simulink model "dynamicDecouplingControl"  (R2017b)
settings: Solver=VariableStepAuto  StartTime=0.0  StopTime=time  RelTol=1e-3
values from neighbouring files (symbols this model uses):
  Kp = eye(2)    [runDynamic.m]    (also in runStatic.m)
  Kv = eye(2)    [runDynamic.m]
  L = 0.13    [runDynamic.m]    (also in runLyapunov.m; runStatic.m)
  L_controller = 0.13    [runDynamic.m]    (also in runLyapunov.m = 0.143; runStatic.m)
  R = 2    [runDynamic.m]    (also in runLyapunov.m; runStatic.m)
  r = 0.1    [runDynamic.m]    (also in runLyapunov.m; runStatic.m)
  r_controller = 0.1    [runDynamic.m]    (also in runLyapunov.m; runStatic.m)
  satMax = inf    [runDynamic.m]    (also in runLyapunov.m; runStatic.m)
  satMin = -inf    [runDynamic.m]    (also in runLyapunov.m; runStatic.m)
  wd = 0.5    [runDynamic.m]    (also in runLyapunov.m; runStatic.m)
  Xi = [2.3; 0; pi]    [runDynamic.m]    (also in runLyapunov.m; runStatic.m)
settings Model: Creator=yleni  LastModifiedBy=yleni

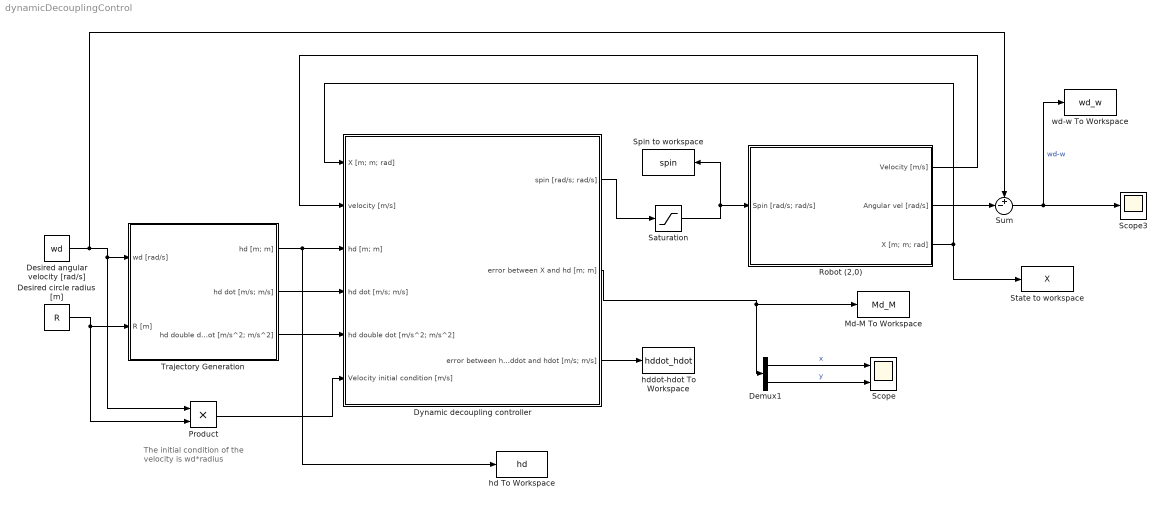
== system dynamicDecouplingControl ==
  note: The initial condition of the
      | velocity is wd*radius
  Demux1 : Demux  Outputs=2
  Desired angular velocity [rad/s] : Constant  Value=wd
  Desired circle radius [m] : Constant  Value=R
  Dynamic decoupling controller : Subsystem  mask{Kp=Kp, Kv=Kv, L=L_controller, r=r_controller}
      mask prompts: Kp "Gain position control law"; Kv "Gain velocity control law"; L "Distance from the wheel to the robot frame center [m]"; r "Wheel radius [m]"
      settings: MinAlgLoopOccurrences=on
  Md-M To Workspace : ToWorkspace  VariableName=Md_M  SampleTime=-1
      settings: Save2DSignal=2-D array (concatenate along first dimension)
  Product : Product
  Robot (2,0) : Subsystem  mask{r=r, L=L, Xstart=Xi}
      mask prompts: r "Wheel radius [m]"; L "Distance from the wheel to the robot frame center [m]"; Xstart "Initial conditions [m; m; rad]"
  Saturation : Saturate  UpperLimit=satMax  LowerLimit=satMin
  Scope : Scope  NumInputPorts=2
  Scope3 : Scope
  Spin to workspace : ToWorkspace  VariableName=spin  SampleTime=-1
      settings: Save2DSignal=2-D array (concatenate along first dimension)
  State to workspace : ToWorkspace  VariableName=X  SampleTime=-1
      settings: Save2DSignal=2-D array (concatenate along first dimension)
  Sum : Sum  Inputs=+-|
  Trajectory Generation : Subsystem
  hd To Workspace : ToWorkspace  VariableName=hd  SampleTime=-1
      settings: Save2DSignal=2-D array (concatenate along first dimension)
  hddot-hdot To Workspace : ToWorkspace  VariableName=hddot_hdot  SampleTime=-1
      settings: Save2DSignal=2-D array (concatenate along first dimension)
  wd-w To Workspace : ToWorkspace  VariableName=wd_w  SampleTime=-1
      settings: Save2DSignal=2-D array (concatenate along first dimension)
  wires:
  Robot (2,0)/3(X [m; m; rad]) -> State to workspace/1, Dynamic decoupling controller/1(X [m; m; rad])
  Desired circle radius [m]/1 -> Product/2, Trajectory Generation/2(R [m])
  Trajectory Generation/1(hd [m; m]) -> hd To Workspace/1, Dynamic decoupling controller/3(hd [m; m])
  Trajectory Generation/2(hd dot [m/s; m/s]) -> Dynamic decoupling controller/4(hd dot [m/s; m/s])
  Trajectory Generation/3(hd double dot [m/s^2; m/s^2]) -> Dynamic decoupling controller/5(hd double dot [m/s^2; m/s^2])
  Dynamic decoupling controller/1(spin [rad/s; rad/s]) -> Saturation/1
  Product/1 -> Dynamic decoupling controller/6(Velocity initial condition [m/s])
  Demux1/2 -> Scope/2  "y"
  Dynamic decoupling controller/2(error between X and hd [m; m]) -> Md-M To Workspace/1, Demux1/1
  Demux1/1 -> Scope/1  "x"
  Desired angular velocity [rad/s]/1 -> Sum/1, Product/1, Trajectory Generation/1(wd [rad/s])
  Sum/1 -> wd-w To Workspace/1, Scope3/1  "wd-w"
  Robot (2,0)/2(Angular vel [rad/s]) -> Sum/2
  Saturation/1 -> Spin to workspace/1, Robot (2,0)/1(Spin [rad/s; rad/s])
  Dynamic decoupling controller/3(error between hddot and hdot [m/s; m/s]) -> hddot-hdot To Workspace/1
  Robot (2,0)/1(Velocity [m/s]) -> Dynamic decoupling controller/2(velocity [m/s])

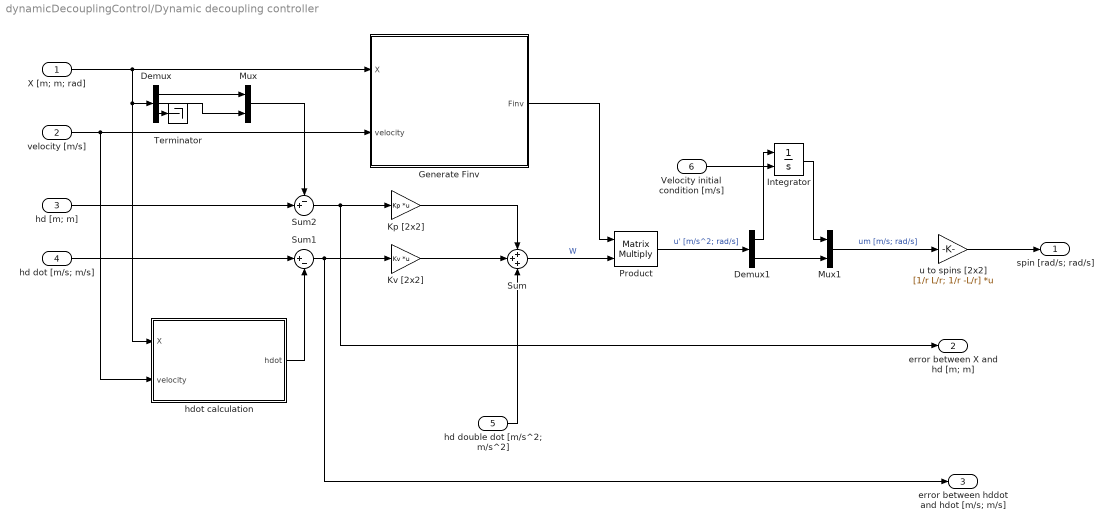
== system dynamicDecouplingControl/Dynamic decoupling controller ==
  X [m; m; rad] : Inport
  velocity [m/s] : Inport  Port=2
  hd [m; m] : Inport  Port=3
  hd dot [m/s; m/s] : Inport  Port=4
  hd double dot [m/s^2; m/s^2] : Inport  Port=5
  Velocity initial condition [m/s] : Inport  Port=6
  Demux : Demux  Outputs=3
  Demux1 : Demux  Outputs=2
  Generate Finv : MATLAB Function  TreatAsAtomicUnit=on
  Integrator : Integrator  InitialConditionSource=external
  Kp [2x2] : Gain  Gain=Kp  Multiplication=Matrix(K*u)
  Kv [2x2] : Gain  Gain=Kv  Multiplication=Matrix(K*u)
  Mux : Mux  Inputs=2
  Mux1 : Mux  Inputs=2
  Product : Product  Multiplication=Matrix(*)
  Sum : Sum  Inputs=+++
  Sum1 : Sum  Inputs=|+-
  Sum2 : Sum  Inputs=-+|
  Terminator : Terminator
  hdot calculation : MATLAB Function  TreatAsAtomicUnit=on
  u to spins [2x2] : Gain  Gain=[1/r L/r; 1/r -L/r]  Multiplication=Matrix(K*u)
  spin [rad/s; rad/s] : Outport
  error between X and hd [m; m] : Outport  Port=2
  error between hddot and hdot [m/s; m/s] : Outport  Port=3
  wires:
  Kv [2x2]/1 -> Sum/2
  Kp [2x2]/1 -> Sum/1
  Generate Finv/1(Finv) -> Product/1
  Sum/1 -> Product/2  "W"
  X [m; m; rad]/1 -> hdot calculation/1(X), Demux/1, Generate Finv/1(X)
  hd double dot [m/s^2; m/s^2]/1 -> Sum/3
  Sum1/1 -> error between hddot and hdot [m/s; m/s]/1, Kv [2x2]/1
  hd dot [m/s; m/s]/1 -> Sum1/1
  Sum2/1 -> error between X and hd [m; m]/1, Kp [2x2]/1
  hd [m; m]/1 -> Sum2/2
  Demux/1 -> Mux/1
  Demux/2 -> Mux/2
  Mux/1 -> Sum2/1
  hdot calculation/1(hdot) -> Sum1/2
  Product/1 -> Demux1/1  "u' [m/s^2; rad/s]"
  Demux1/2 -> Mux1/2
  Mux1/1 -> u to spins [2x2]/1  "um [m/s; rad/s]"
  u to spins [2x2]/1 -> spin [rad/s; rad/s]/1
  Demux/3 -> Terminator/1
  Velocity initial condition [m/s]/1 -> Integrator/2
  Integrator/1 -> Mux1/1
  velocity [m/s]/1 -> hdot calculation/2(velocity), Generate Finv/2(velocity)
  Demux1/1 -> Integrator/1

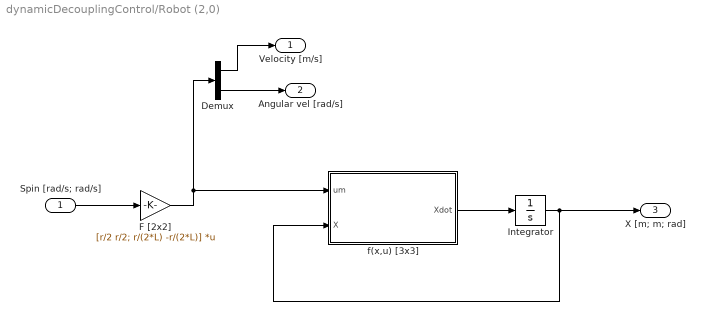
== system dynamicDecouplingControl/Robot (2,0) ==
  Spin [rad/s; rad/s] : Inport
  Demux : Demux  Outputs=2
  F [2x2] : Gain  Gain=[r/2 r/2; r/(2*L) -r/(2*L)]  Multiplication=Matrix(K*u)
  Integrator : Integrator  InitialCondition=Xstart
  f(x,u) [3x3] : MATLAB Function  TreatAsAtomicUnit=on
  Velocity [m/s] : Outport
  Angular vel [rad/s] : Outport  Port=2
  X [m; m; rad] : Outport  Port=3
  wires:
  f(x,u) [3x3]/1(Xdot) -> Integrator/1
  F [2x2]/1 -> f(x,u) [3x3]/1(um), Demux/1
  Demux/2 -> Angular vel [rad/s]/1
  Demux/1 -> Velocity [m/s]/1
  Integrator/1 -> X [m; m; rad]/1, f(x,u) [3x3]/2(X)
  Spin [rad/s; rad/s]/1 -> F [2x2]/1

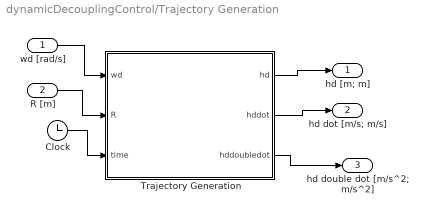
== system dynamicDecouplingControl/Trajectory Generation ==
  wd [rad/s] : Inport
  R [m] : Inport  Port=2
  Clock : Clock
  Trajectory Generation : MATLAB Function  TreatAsAtomicUnit=on
  hd [m; m] : Outport
  hd dot [m/s; m/s] : Outport  Port=2
  hd double dot [m/s^2; m/s^2] : Outport  Port=3
  wires:
  wd [rad/s]/1 -> Trajectory Generation/1(wd)
  Trajectory Generation/2(hddot) -> hd dot [m/s; m/s]/1
  R [m]/1 -> Trajectory Generation/2(R)
  Trajectory Generation/1(hd) -> hd [m; m]/1
  Clock/1 -> Trajectory Generation/3(time)
  Trajectory Generation/3(hddoubledot) -> hd double dot [m/s^2; m/s^2]/1

== matlab function dynamicDecouplingControl/Dynamic decoupling controller/Generate Finv ==
  data: X input; Finv output; velocity input
function Finv = generateFinv(X, velocity)

F = [cos(X(3)) -velocity*sin(X(3)); sin(X(3)) velocity*cos(X(3))];
Finv = inv(F);

== matlab function dynamicDecouplingControl/Robot (2,0)/f(x,u) [3x3] ==
  data: um input; Xdot output; X input
function Xdot  = evolutionModel(um, X)

Xdot = zeros(3,1);
Xdot(1) = um(1) * cos(X(3));
Xdot(2) = um(1) * sin(X(3));
Xdot(3) = um(2);

== matlab function dynamicDecouplingControl/Trajectory Generation/Trajectory Generation ==
  data: wd input; hd output; R input; time input; hddot output; hddoubledot output
function [hd, hddot, hddoubledot] = trajectoryGeneration(wd, R, time)

hd = [R*cos(wd*time); R*sin(wd*time)];

hddot = [-R*sin(wd*time)*wd; R*cos(wd*time)*wd];

hddoubledot = [-R*cos(wd*time)*wd*wd; -R*sin(wd*time)*wd*wd];

== matlab function dynamicDecouplingControl/Dynamic decoupling controller/hdot calculation ==
  data: X input; hdot output; velocity input
function hdot = calculatehdot(X, velocity)

hdot = [velocity*cos(X(3)); velocity*sin(X(3))];
